simulink model "demoDPThrusterModels"  (R2020a)
settings: Solver=ode45  StartTime=0.0  StopTime=200  RelTol=1e-3  EnableMultiTasking=on
undefined symbols (not defined in the file): slcm
libraries: mssSimulink x2, simulink_extras x2, simulink x1
settings Model: Creator=thor  LastModifiedBy=thor
settings DataIOCC: LimitDataPoints=on  SaveFormat=Array  SignalLoggingSaveFormat=ModelDataLogs  ReturnWorkspaceOutputs=off  SignalLoggingName=sigsOut
settings OptimizationCC: InitFltsAndDblsToZero=on  LifeSpan=inf
settings DebuggingCC: SaveWithParameterizedLinksMsg=none  UnderspecifiedInitializationDetection=Classic  MergeDetectMultiDrivingBlocksExec=none  SignalResolutionControl=TryResolveAllWithWarning  MultiTaskDSMMsg=warning  MultiTaskCondExecSysMsg=none  FcnCallInpInsideContextMsg=warning  SFUnexpectedBacktrackingDiag=warning  SFNoUnconditionalDefaultTransitionDiag=warning  SFExecutionAtInitializationDiag=none  ArithmeticOperatorsInVariantConditions=warning
settings HardwareCC: ProdBitPerPointer=32  ProdBitPerSizeT=32  ProdBitPerPtrDiffT=32  ProdLargestAtomicFloat=None  ProdIntDivRoundTo=Undefined  ProdEndianess=Unspecified  ProdWordSize=32  ProdHWDeviceType=32-bit Generic  TargetUnknown=on
settings ModelReferenceCC: PropagateSignalLabelsOutOfModel=off
settings CodeAppCC: StateflowObjectComments=on
settings GRTTargetCC: TargetFcnLib=ansi_tfl_tmw.mat  TargetLangStandard=C89/C90 (ANSI)  ModelReferenceCompliant=off  CombineOutputUpdateFcns=off  MatFileLogging=off  GRTInterface=on
settings ConfigComp: CovMetricSettings=dw  CovHtmlReporting=on  CovSaveCumulativeToWorkspaceVar=on  CovSaveSingleToWorkspaceVar=on

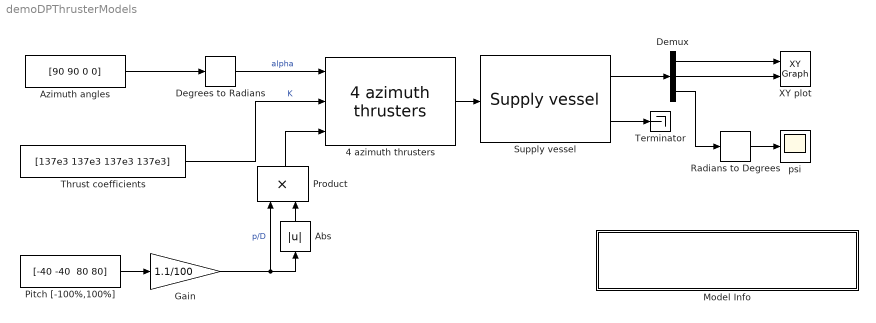
== system demoDPThrusterModels ==
  "4 azimuth thrusters " : mssSimulink/Modelling/Propulsion/Actuator Configuration/4 azimuth thrusters  SystemSampleTime=-1  Latency=0  AutoFrameSizeCalculation=off
  Abs : Abs  SaturateOnIntegerOverflow=on
  Azimuth angles : Constant  Value=[90 90 0 0]
  Degrees to Radians : simulink_extras/Transformations/Degrees to Radians
  Demux : Demux  Outputs=3
      settings: DisplayOption=none
  Gain : Gain  Gain=1.1/100  SaturateOnIntegerOverflow=on  OutDataTypeStr=Inherit: Same as input  ParamDataTypeStr=Inherit: Same as input
  Model Info : Subsystem  LoadFcn=slcm LoadBlock;  InitFcn=slcm('UpdateAllCMBlocksInThisModelInit')  mask(CMBlock){InitialSaveTempField=, InitialBlockCM=None, BlockCM=None, Frame=on, SaveTempField=, DisplayStringWithTags=|, MaskDisplayString=Demo showing how 4 azimuth thrusters\ncan be configured for a supply vessel\nAuthor: Thor I. Fossen\nThu Mar 04 19:38:13 2021, HorizontalTextAlignment=Left, LeftAlignmentValue=0.02, SourceBlockDiagram=demothr, TagMaxNumber=20, CMTag1=, CMTag2=, CMTag3=, CMTag4=, CMTag5=, CMTag6=, CMTag7=, CMTag8=, CMTag9=, CMTag10=, CMTag11=, CMTag12=, CMTag13=, CMTag14=, CMTag15=, CMTag16=, CMTag17=, CMTag18=, CMTag19=, CMTag20=}
      mask DisplayStringWithTags=|
      | Demo showing how 4 azimuth thrusters
      | can be configured for a supply vessel
      | Author: Thor I. Fossen
      | %<LastModificationDate>
      mask help: This block allows revision control information to be displayed within the model.
      settings: CopyFcn=slcm CopyBlock;  DeleteFcn=slcm Cancel;  PostSaveFcn=slcm('UpdateAllCMBlocksInThisModel')  NameChangeFcn=slcm Rename;  OpenFcn=slcm
      mask Display: text(str2num(LeftAlignmentValue), 0.5, MaskDisplayString, 'HorizontalAlignment', HorizontalTextAlignment)
  Pitch [-100%,100%] : Constant  Value="[-40 -40  80 80]"
  Product : Product  SaturateOnIntegerOverflow=on  OutDataTypeStr=Inherit: Same as first input
  Radians to Degrees : simulink_extras/Transformations/Radians to Degrees
  "Supply vessel " : mssSimulink/Marine craft models/Supply vessel  D=[5.0242e4 0 0; 0 2.7229e5 -4.3933e6; 0 -4.3933e6 4.1894e8]  Minv=inv( [5.3122e6 0 0; 0 8.2831e6 0; 0 0 3.7454e9] )
  Terminator : Terminator
  Thrust coefficients : Constant  Value=[137e3 137e3 137e3 137e3]
  XY plot : simulink/Sinks/XY Graph  xmin=-500  xmax=500  ymin=-500  ymax=500  st=-1
  psi : Scope
  wires:
  "4 azimuth thrusters "/1 -> "Supply vessel "/1
  "Supply vessel "/1 -> Demux/1
  Demux/1 -> XY plot/1
  Demux/2 -> XY plot/2
  "Supply vessel "/2 -> Terminator/1
  Degrees to Radians/1 -> "4 azimuth thrusters "/1  "alpha"
  Thrust coefficients/1 -> "4 azimuth thrusters "/2  "K"
  Pitch [-100%,100%]/1 -> Gain/1
  Abs/1 -> Product/2
  Gain/1 -> Product/1, Abs/1  "p/D"
  Product/1 -> "4 azimuth thrusters "/3
  Demux/3 -> Radians to Degrees/1
  Radians to Degrees/1 -> psi/1
  Azimuth angles/1 -> Degrees to Radians/1

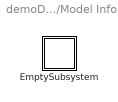
== system demoDPThrusterModels/Model Info ==
  EmptySubsystem : Subsystem

== system demoDPThrusterModels/Model Info/EmptySubsystem ==
